simulink model "Test_N6"  (R2020b)
settings: Solver=ode3  StartTime=0.0  StopTime=inf  FixedStep=0.05  RelTol=1e-3
libraries: XBotBlockToolbox x2

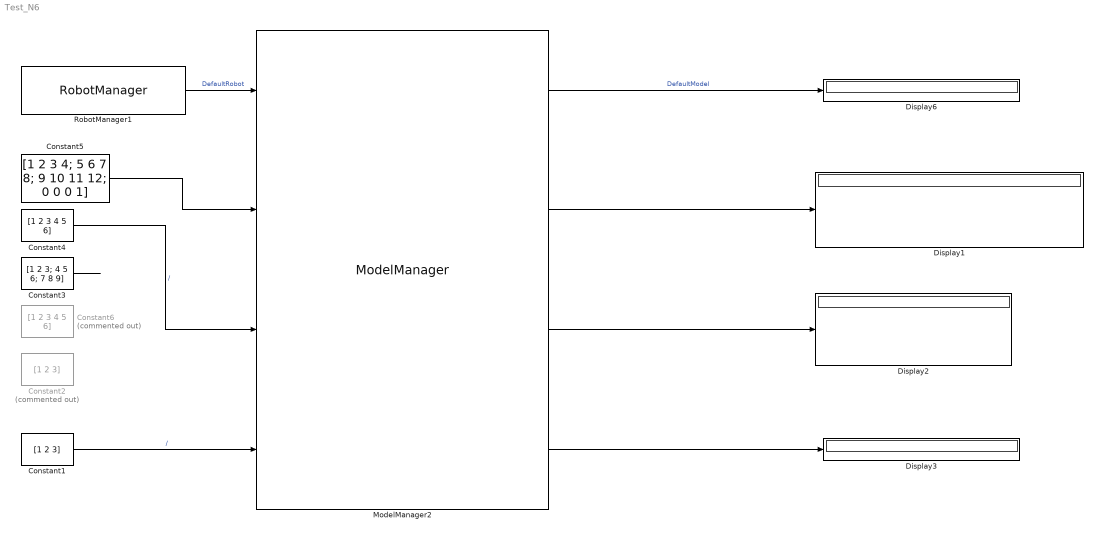
== system Test_N6 ==
  Constant1 : Constant  Value=[1 2 3]
  Constant2 : Constant  Commented=on  Value=[1 2 3]
  Constant3 : Constant  Value=[1 2 3; 4 5 6; 7 8 9]
  Constant4 : Constant  Value=[1 2 3 4 5 6]
  Constant5 : Constant  Value=[1 2 3 4; 5 6 7 8; 9 10 11 12; 0 0 0 1]
  Constant6 : Constant  Commented=on  Value=[1 2 3 4 5 6]
  Display{1..3,6} (4 alike) : Display
  ModelManager2 : XBotBlockToolbox/ModelManager  ModelName=DefaultModel  RobotName=DefaultRobot  UseExtModel=Off  SyncWithRobot=On  GetFloatingBaseList={ 'Pose', 'Twist' }  SetFloatingBaseComponent=State  GravityRequest=Both  ReadingsList={}  MechanicalLimitsList={}  MechanicalLimitsCheck=Off  MechanicalLimitsEnforce=Off  SensorList={}  ReferencesList={}  OldModelName=DefaultModel
  RobotManager1 : XBotBlockToolbox/RobotManager  RobotName=DefaultRobot  ModelName=DefaultModel  UseExtRobot=Off  SyncWithModel=Off  ReadingsList={}  MechanicalLimitsList={}  MechanicalLimitsCheck=Off  MechanicalLimitsEnforce=Off  SensorList={}  ReferencesList={}  OldRobotName=DefaultRobot
  wires:
  RobotManager1/1 -> ModelManager2/1  "DefaultRobot"
  ModelManager2/1 -> Display6/1  "DefaultModel"
  ModelManager2/2 -> Display1/1
  ModelManager2/3 -> Display2/1
  ModelManager2/4 -> Display3/1
  Constant3/1 -> ?
  Constant5/1 -> ModelManager2/2
  Constant4/1 -> ModelManager2/3  "/"
  Constant1/1 -> ModelManager2/4  "/"
